simulink model "snap2_f_200msps_64i_4096c_test"  (R2019a)
settings: Solver=VariableStepDiscrete  StartTime=0.0  StopTime=10.0  RelTol=1e-3
libraries: xbsIndex_r4 x8040, casper_library_misc x13, xps_library x6, casper_library_delays x4, casper_library_sources x4, casper_library_reorder x2
(part 1 of 84)
settings Model: ModifiedComment=jackh -- Sun May 10 19:52:36 2020 -- Version 1.426  Creator=mdexter  LastModifiedBy=jackh
settings Model: ModifiedHistory=|
  | jackh -- Sun May 10 19:52:36 2020 -- Version 1.426
  | 
  | jackh -- Sun May 10 19:42:43 2020 -- Version 1.425
  | 
  | make dest udp port dynamically choosable per-packet
  | 
  | jackh -- Sun May 10 17:04:12 2020 -- Version 1.424
  | 
  | make version 0.1
  | 
  | jackh -- Sun May 10 17:03:03 2020 -- Version 1.423
  | 
  | Reorder pols in chan_reorder block so that pol indexing
  | is pol[n] = nth byte of packet
  | 
  | jackh -- Sun May 10 16:52:32 2020 -- Version 1.422
  | 
  | jackh -- Sun May 10 16:08:00 2020 -- Version 1.421
  | 
  | jackh -- Fri May 08 15:06:38 2020 -- Version 1.420
  | 
  | jackh -- Thu May 07 11:32:09 2020 -- Version 1.419
  | 
  | jackh -- Thu May 07 11:18:16 2020 -- Version 1.418
  | 
  | Remove PFB
  | 
  | jackh -- Tue May 05 14:16:03 2020 -- Version 1.417
  | 
  | Make version 0
  | 
  | jackh -- Tue May 05 14:15:21 2020 -- Version 1.416
  | 
  | replace ADC with zeros
  | 
  | jackh -- Tue May 05 14:14:14 2020 -- Version 1.415
  | 
  | Make test design, which is clocked from sys clock and has no ADC
  | 
  | jackh -- Tue May 05 13:29:10 2020 -- Version 1.414
  | 
  | jackh -- Fri May 01 15:26:24 2020 -- Version 1.413
  | 
  | Use sys_clk for testing
  | 
  | jackh -- Fri May 01 15:14:39 2020 -- Version 1.412
  | 
  | Rename 1Gbe core so it is alphabetically first
  | 
  | jackh -- Fri May 01 15:11:49 2020 -- Version 1.411
  | 
  | jackh -- Fri May 01 11:15:12 2020 -- Version 1.410
  | 
  | Change 40gbe core enable so that software enable state can only change immediately after an EOF
  | 
  | jackh -- Fri Apr 24 17:52:32 2020 -- Version 1.409
  | 
  | jackh -- Fri Apr 24 17:51:51 2020 -- Version 1.408
  | 
  | jackh -- Fri Apr 24 17:50:48 2020 -- Version 1.407
  | 
  | jackh -- Fri Apr 24 17:48:49 2020 -- Version 1.406
  | 
  | make packetizer simpler
  | 
  | jackh -- Fri Apr 24 16:17:31 2020 -- Version 1.405
  | 
  | ass max_delay register to delay core
  | 
  | jackh -- Fri Apr 24 16:14:09 2020 -- Version 1.404
  | 
  | jackh -- Fri Apr 24 16:12:03 2020 -- Version 1.403
  | 
  | update eq_tvg to single bram
  | 
  | jackh -- Fri Apr 24 16:08:40 2020 -- Version 1.402
  | 
  | jackh -- Thu Apr 09 09:24:59 2020 -- Version 1.401
  | 
  | make delays 8k long
  | 
  | jackh -- Mon Mar 30 21:41:54 2020 -- Version 1.400
  | 
  | add 1gbe core
  | 
  | jackh -- Sat Mar 14 14:05:43 2020 -- Version 1.399
  | 
  | jackh -- Wed Feb 19 18:48:51 2020 -- Version 1.398
  | 
  | jackh -- Wed Feb 19 18:31:56 2020 -- Version 1.397
  | 
  | jackh -- Wed Feb 19 18:25:06 2020 -- Version 1.396
  | 
  | jackh -- Wed Feb 19 17:10:23 2020 -- Version 1.395
  | 
  | add back in reorders in pfb (having fixed mlib_devel)
  | 
  | jackh -- Tue Feb 18 17:39:49 2020 -- Version 1.394
  | 
  | 10 bitify
  | 
  | jackh -- Tue Feb 18 17:31:23 2020 -- Version 1.393
  | 
  | update_casper_blocks
  | 
  | jackh -- Fri Jan 24 08:04:16 2020 -- Version 1.392
  | replace ADC with sw regs to try and compile for SNAP2
  | 
  | jackh -- Wed Jan 08 08:41:40 2020 -- Version 1.391
  | 
  | 
  | jackh -- Wed Jan 08 08:26:20 2020 -- Version 1.390
  | 
  | 
  | jackh -- Wed Jan 08 08:24:50 2020 -- Version 1.389
  | 
  | 
  | jackh -- Wed Jan 08 08:23:40 2020 -- Version 1.388
  | 
  | 
  | jackh -- Wed Jan 08 08:22:29 2020 -- Version 1.387
  | update platform to SNAP2
  | 
  | jackh -- Wed Jan 08 08:21:36 2020 -- Version 1.386
  | 
  | 
  | jackh -- Wed Jan 08 08:21:09 2020 -- Version 1.385
  | Update internal cross-corr block
  | 
  | jackh -- Wed Jan 08 07:50:59 2020 -- Version 1.384
  | 
  | 
  | jackh -- Wed Jan 08 07:48:46 2020 -- Version 1.383
  | 
  | 
  | jackh -- Wed Jan 08 07:45:47 2020 -- Version 1.382
  | 
  | 
  | jackh -- Wed Jan 08 07:44:03 2020 -- Version 1.381
  | 
  | 
  | jackh -- Wed Jan 08 07:41:17 2020 -- Version 1.380
  | 
  | 
  | jackh -- Wed Jan 08 07:35:58 2020 -- Version 1.379
  | 
  | 
  | jackh -- Wed Jan 08 07:33:51 2020 -- Version 1.378
  | 
  | 
  | jackh -- Wed Jan 08 07:29:30 2020 -- Version 1.377
  | 
  | 
  | jackh -- Wed Jan 08 07:24:27 2020 -- Version 1.376
  | 1st pass fuilly updated to LWA spec
  | 
  | jackh -- Tue Jan 07 10:50:49 2020 -- Version 1.375
  | 
  | 
  | jackh -- Tue Jan 07 10:38:05 2020 -- Version 1.374
  | EQ tvg & FFT updated for 64 inputs
  | 
  | jackh -- Tue Jan 07 10:18:18 2020 -- Version 1.373
  | 
  | 
  | jackh -- Tue Jan 07 10:12:36 2020 -- Version 1.372
  | update FFT
  | 
  | jackh -- Tue Jan 07 09:22:52 2020 -- Version 1.371
  | update FFT core (currently only doing 1/4 of the necessary work)
  | 
  | jackh -- Tue Jan 07 07:40:39 2020 -- Version 1.370
  | Make 64-input. Only corrected up to FFT inputs
  | 
  | jackh -- Tue Jan 07 06:33:25 2020 -- Version 1.369
  | Save a version for LWA expansion project.
  | 
  | jackh -- Sun Oct 27 09:17:26 2019 -- Version 1.368
  | compiled
  | 
  | jackh -- Sun Oct 27 07:24:12 2019 -- Version 1.367
  | remove registering of reorder outputs
  | 
  | jackh -- Sun Oct 27 07:22:37 2019 -- Version 1.366
  | change input snapshot to snap only one of 3 inputs
  | 
  | jackh -- Sun Oct 27 03:59:18 2019 -- Version 1.365
  | remove some superfluous registers to improve timing.
  | Reduce snapshot in input block from 1k samples to 512
  | 
  | jackh -- Sun Oct 27 01:46:50 2019 -- Version 1.364
  | Fix FFT shift bitwidth bug
  | 
  | FFT core was expecting a 16-bit shift, but only a 12bit value was sliced from the control register
  | 
  | jackh -- Fri Aug 30 09:22:01 2019 -- Version 1.363
  | compiled
  | 
  | jackh -- Thu Aug 29 17:13:27 2019 -- Version 1.362
  | change delay shift reg to 3 bit addr
  | 
  | jackh -- Thu Aug 29 11:33:13 2019 -- Version 1.361
  | corr fixes
  | 
  | jackh -- Thu Aug 29 11:09:21 2019 -- Version 1.360
  | latency fix in eqtvg
  | 
  | jackh -- Thu Aug 29 10:02:04 2019 -- Version 1.359
  | compiled
  | 
  | jackh -- Wed Aug 28 15:31:00 2019 -- Version 1.358
  | bump to version 1.3
  | 
  | jackh -- Wed Aug 28 15:26:18 2019 -- Version 1.357
  | change quantization to saturate.
  | Change coefficients to 16_5 (was 16_6)
  | 
  | jackh -- Wed Aug 28 14:17:28 2019 -- Version 1.356
  | remove debugging snapshots hidden in corr vaccs
  | 
  | jackh -- Fri Aug 23 15:01:55 2019 -- Version 1.355
  | compiled
  | 
  | jackh -- Fri Aug 23 10:43:05 2019 -- Version 1.354
  | add snapshot in input block
  | 
  | jackh -- Thu Aug 22 17:13:50 2019 -- Version 1.353
  | fix to eqtvg ram depths
  | 
  | jackh -- Thu Aug 22 15:23:14 2019 -- Version 1.352
  | bump version to 1.2
  | 
  | jackh -- Thu Aug 22 15:22:39 2019 -- Version 1.351
  | Force pairs of pols to have same random number generator to save resources
  | 
  | jackh -- Thu Aug 22 15:19:21 2019 -- Version 1.350
  | rotator channel index counter fixes
  | 
  | eq tvg split bram into 3 (so we can have 6 channels, not 8)
  | 
  | jackh -- Thu Aug 22 12:01:44 2019 -- Version 1.349
  | 
  | 
  | jackh -- Thu Aug 22 12:01:21 2019 -- Version 1.348
  | Changes to rotator precision
  | 
  | jackh -- Tue Aug 20 19:46:09 2019 -- Version 1.347
  | compiled
  | 
  | jackh -- Tue Aug 20 16:55:38 2019 -- Version 1.346
  | increase minimum walsh period to 2**18 fpga clocks (was 2**13)
  | 
  | jackh -- Tue Aug 20 16:40:34 2019 -- Version 1.345
  | 
  | 
  | jackh -- Tue Aug 20 16:15:18 2019 -- Version 1.344
  | bump version to 1.1
  | 
  | jackh -- Tue Aug 20 16:14:49 2019 -- Version 1.343
  | add global enables to phase switch mod/demod to make software easier
  | 
  | jackh -- Mon Aug 19 17:54:23 2019 -- Version 1.342
  | compiled
  | 
  | jackh -- Thu Aug 01 11:53:22 2019 -- Version 1.341
  | make programmable sync delay tolerate delay=0
  | 
  | jackh -- Wed Jul 31 13:49:54 2019 -- Version 1.340
  | comment out corr->rms
  | 
  | jackh -- Mon Jul 29 17:05:34 2019 -- Version 1.339
  | delete corr rms block (not currently enough ram)
  | 
  | jackh -- Mon Jul 29 17:03:29 2019 -- Version 1.338
  | Add version block
  | 
  | jackh -- Mon Jul 29 16:58:22 2019 -- Version 1.337
  | make sync in have a programmable delay
  | Solves 2 problems:
  | 
  | 1) Can start integrations at arbitrary times (good for LST alignment)
  | 2) Can start a 16 second integration chunk on an arbitrary time boundary (needed to avoid the downstream correlator having 16 second start / stop granularity)
  | 
  | jackh -- Mon Jul 29 16:50:03 2019 -- Version 1.336
  | update phasor to 24-bits
  | 
  | jackh -- Sat May 11 17:48:41 2019 -- Version 1.335
  | 
  | 
  | jackh -- Sat May 11 17:46:07 2019 -- Version 1.334
  | 
  | 
  | jackh -- Sat May 11 17:45:44 2019 -- Version 1.333
  | 
  | 
  | jackh -- Sat May 11 17:40:04 2019 -- Version 1.332
  | 
  | 
  | jackh -- Sat May 11 17:36:59 2019 -- Version 1.331
  | add vacc for autocorrs @ 16 bit resolution
  | 
  | deepthi -- Sun Oct 28 15:16:19 2018 -- Version 1.330
  | 
  | 
  | deepthi -- Sat Oct 27 18:45:54 2018 -- Version 1.329
  | 
  | packetizer: Added an 'and' block that holds new_packet signal in high until the first sync.
  | 
  | deepthi -- Sat Oct 27 17:33:32 2018 -- Version 1.328
  | 
  | 1. Change edge_detect location in sync block
  | 
  | deepthi -- Sat Oct 20 22:13:43 2018 -- Version 1.327
  | 
  | 1. Add edge detect to software reg and gpio input in sync block.
  | 
  | 2. Add new corr block with max hold functionality.
  | 
  | jackh -- Tue Oct 09 20:34:13 2018 -- Version 1.326
  | recompile with pmbus_alert register
  | 
  | jackh -- Thu Jul 12 10:55:28 2018 -- Version 1.325
  | 
  | 
  | jackh -- Wed Jul 11 17:20:51 2018 -- Version 1.324
  | syntax
  | 
  | jackh -- Wed Jul 11 17:16:24 2018 -- Version 1.323
  | increase resolution of phase rotator bram.
  | 
  | jackh -- Wed Jul 11 17:10:41 2018 -- Version 1.322
  | 
  | 
  | jackh -- Tue Jul 10 16:08:30 2018 -- Version 1.321
  | scramble rotator channel multiplers to match PFB output order (hopefully)
  | 
  | jackh -- Tue Jul 10 15:51:56 2018 -- Version 1.320
  | 
  | 
  | jackh -- Tue Jul 10 13:37:24 2018 -- Version 1.319
  | fix off-by-one in slicing of mcnt counter, which was having the effect of duplicating mcnts in headers
  | 
  | jackh -- Sat Jul 07 14:17:05 2018 -- Version 1.318
  | compiled
  | 
  | jackh -- Fri Jul 06 10:33:47 2018 -- Version 1.317
  | fix bitbashing to rotator phase addresses
  | 
  | jackh -- Fri Jul 06 10:17:15 2018 -- Version 1.316
  | Add mux to enable / disable rotator
  | 
  | jackh -- Thu Jul 05 17:21:10 2018 -- Version 1.315
  | make some delays behavioural
  | 
  | jackh -- Thu Jul 05 14:48:28 2018 -- Version 1.314
  | 
  | 
  | jackh -- Thu Jul 05 14:46:13 2018 -- Version 1.313
  | 
  | 
  | jackh -- Thu Jul 05 14:43:36 2018 -- Version 1.312
  | 
  | 
  | jackh -- Thu Jul 05 14:40:00 2018 -- Version 1.311
  | 
  | 
  | jackh -- Thu Jul 05 14:36:19 2018 -- Version 1.310
  | 
  | 
  | jackh -- Thu Jul 05 14:26:16 2018 -- Version 1.309
  | integrate rotator into pipeline
  | 
  | jackh -- Thu Jul 05 14:20:20 2018 -- Version 1.308
  | 
  | create phase-rotation block
  | 
  | deepthi -- Thu Jun 07 09:24:03 2018 -- Version 1.307
  | 
  | Replaced the corr block.
  | 
  | deepthi -- Wed Jun 06 12:07:26 2018 -- Version 1.306
  | 
  | 
  | deepthi -- Tue Jun 05 17:46:17 2018 -- Version 1.305
  | 
  | Replaced the corr block with the tested version
  | 
  | deepthi -- Sat May 12 19:11:02 2018 -- Version 1.304
  | 
  | Changed time counter to increment between even/odd banks
  | 
  | deepthi -- Sat May 12 19:06:34 2018 -- Version 1.303
  | 
  | changed timing of eof, valid, data and headers
  | 
  | deepthi -- Mon May 07 23:03:07 2018 -- Version 1.302
  | 
  | 
  | deepthi -- Mon May 07 00:31:44 2018 -- Version 1.301
  | 
  | 
  | deepthi -- Fri May 04 20:13:43 2018 -- Version 1.300
  | 
  | Reduced width sliced from time_ctr
  | 
  | deepthi -- Fri May 04 19:47:57 2018 -- Version 1.299
  | 
  | Added delay to header and ip signals to account for pulse_ext on valid.
  | 
  | deepthi -- Fri May 04 19:23:23 2018 -- Version 1.298
  | 
  | 
  | deepthi -- Thu May 03 16:58:39 2018 -- Version 1.297
  | 
  | 1. Added delays to eof and dest_ip  to account for pulse_ext in valid.
  | 
  | 2. Changed eth_sw expected packet length to include header.
  | 
  | jackh -- Tue May 01 20:38:09 2018 -- Version 1.296
  | compiled
  | 
  | jackh -- Tue May 01 17:49:38 2018 -- Version 1.295
  | Fix to packetizer valid generation, to take into account the 3 (one per antenna) blocks of valid data in each stream of 512 channels
  | 
  | jackh -- Tue May 01 16:49:02 2018 -- Version 1.294
  | make channel selection bram 32-bits wide.
  | 
  | Remove GPU-packing mux / swreg
  | 
  | jackh -- Tue May 01 14:24:16 2018 -- Version 1.293
  | 
  | 
  | jackh -- Tue May 01 14:20:01 2018 -- Version 1.292
  | update chan reorderer
  | 
  | jackh -- Tue May 01 11:43:41 2018 -- Version 1.291
  | compiled
  | 
  | jackh -- Tue May 01 09:44:03 2018 -- Version 1.290
  | 
  | 
  | jackh -- Tue May 01 09:43:34 2018 -- Version 1.289
  | use bram for eq fft descramble map
  | 
  | jackh -- Tue May 01 09:40:26 2018 -- Version 1.288
  | change architecture of corr block -- now stores desired antennas in bram, rather than using a delay tree
  | 
  | jackh -- Mon Apr 30 20:21:35 2018 -- Version 1.287
  | 
  | 
  | jackh -- Mon Apr 30 20:18:20 2018 -- Version 1.286
  | 
  | 
  | jackh -- Mon Apr 30 20:15:51 2018 -- Version 1.285
  | compensate for FFT scrambling in EQ block. Descramble FFT post-requantization in this block
  | 
  | jackh -- Mon Apr 30 19:27:42 2018 -- Version 1.284
  | plausibility pass on corr block
  | 
  | jackh -- Mon Apr 30 12:16:47 2018 -- Version 1.283
  | 
  | 
  | jackh -- Mon Apr 30 12:14:25 2018 -- Version 1.282
  | store chan_reorder reorder map in bram
  | 
  | jackh -- Mon Apr 30 12:05:02 2018 -- Version 1.281
  | remove per-antenna histograms -- now get one histogram with multiplexed input
  | 
  | jackh -- Sun Apr 29 15:50:16 2018 -- Version 1.280
  | 
  | 
  | jackh -- Sun Apr 29 15:37:38 2018 -- Version 1.279
  | 
  | 
  | jackh -- Sun Apr 29 15:27:38 2018 -- Version 1.278
  | First pass packetizer. Regenerate pfb with parameter for serial block inputs
  | 
  | jackh -- Sat Mar 03 12:52:57 2018 -- Version 1.277
  | 
  | 
  | jackh -- Sun Feb 25 12:27:48 2018 -- Version 1.276
  | add pre-pfb reorder
  | 
  | jackh -- Sat Feb 24 13:39:06 2018 -- Version 1.275
  | 
  | jackh -- Sat Feb 24 13:38:40 2018 -- Version 1.274
  | update pfb to 16 inputs
  | 
  | jackh -- Fri Feb 23 18:44:26 2018 -- Version 1.273
  | 
  | 
  | jackh -- Fri Feb 23 18:38:20 2018 -- Version 1.272
  | 
  | 
  | jackh -- Fri Feb 23 17:01:30 2018 -- Version 1.271
  | make fft 8 parallel input
  | 
  | jackh -- Sat Feb 10 13:53:12 2018 -- Version 1.270
  | 
  | 
  | jackh -- Sat Feb 10 13:50:10 2018 -- Version 1.269
  | 
  | 
  | jackh -- Sat Feb 10 13:48:56 2018 -- Version 1.268
  | remove fft preshift
  | 
  | jackh -- Sat Feb 10 13:47:39 2018 -- Version 1.267
  | 
  | 
  | jackh -- Sat Feb 10 13:44:29 2018 -- Version 1.266
  | 
  | 
  | jackh -- Sat Feb 10 13:43:22 2018 -- Version 1.265
  | make delayer dual-pol
  | 
  | jackh -- Sat Feb 10 13:40:59 2018 -- Version 1.264
  | first pass new packet format with no time-based corner turn
  | 
  | jackh -- Fri Feb 09 17:29:05 2018 -- Version 1.263
  | 
  | 
  | jackh -- Fri Feb 09 15:23:03 2018 -- Version 1.262
  | first pass turning everything to 8192 channels
  | 
  | Changed the ants addr to be driven by the same signal that drives chans, ips (used to be driven by ant_tracker).
  | 
  | Removed nants software register that was previously thought to control time stamps (but didn't really)
  | 
  | deepthi -- Wed Jan 31 18:20:45 2018 -- Version 1.261
  | 
  | deepthi -- Mon Jan 29 17:20:36 2018 -- Version 1.260
  | 
  | 
  | deepthi -- Mon Jan 29 17:18:54 2018 -- Version 1.259
  | 
  | 
  | deepthi -- Mon Jan 29 17:18:33 2018 -- Version 1.258
  | 
  | 
  | deepthi -- Mon Jan 29 16:51:19 2018 -- Version 1.257
  | 
  | 
  | deepthi -- Mon Jan 29 16:46:46 2018 -- Version 1.256
  | 
  | 
  | deepthi -- Mon Jan 29 16:37:32 2018 -- Version 1.255
  | 
  | 
  | deepthi -- Mon Jan 29 16:11:03 2018 -- Version 1.254
  | 
  | 
  | deepthi -- Mon Jan 29 15:55:33 2018 -- Version 1.253
  | 
  | 
  | jackh -- Fri Nov 17 19:04:05 2017 -- Version 1.252
  | compiled
  | 
  | jackh -- Wed Nov 15 11:31:03 2017 -- Version 1.251
  | go to 3 corr blocks
  | 
  | jackh -- Tue Nov 14 16:10:40 2017 -- Version 1.250
  | 
  | 
  | jackh -- Tue Nov 14 15:28:37 2017 -- Version 1.249
  | reduce bram use in histogram shared brams
  | 
  | jackh -- Mon Nov 13 18:55:18 2017 -- Version 1.248
  | fix bug in histogram shared bram addr width
  | 
  | jackh -- Fri Nov 10 17:05:56 2017 -- Version 1.247
  | add 4 independent corr subsystems. Add EQ clipping counters
  | 
  | jackh -- Fri Nov 10 14:21:14 2017 -- Version 1.246
  | 
  | 
  | jackh -- Fri Nov 10 14:19:27 2017 -- Version 1.245
  | 
  | 
  | jackh -- Fri Nov 10 11:40:47 2017 -- Version 1.244
  | update to histograms v2
  | 
  | jackh -- Tue Nov 07 22:23:59 2017 -- Version 1.243
  | compiled -- passes eqtvg
  | 
  | jackh -- Tue Nov 07 20:41:00 2017 -- Version 1.242
  | 
  | 
  | jackh -- Tue Nov 07 20:39:30 2017 -- Version 1.241
  | packet header generation fixes
  | 
  | jackh -- Tue Nov 07 17:19:53 2017 -- Version 1.240
  | 
  | 
  | jackh -- Tue Nov 07 17:14:47 2017 -- Version 1.239
  | 
  | 
  | jackh -- Tue Nov 07 17:08:29 2017 -- Version 1.238
  | remove some chan_reorder debug snapshots
  | 
  | jackh -- Tue Nov 07 17:06:39 2017 -- Version 1.237
  | update ps GPIO pins
  | 
  | **** Change packetizer header blocks to can have a separate antenna / ip / chan for each packet. This is for the nants > 3 simulation modes. This will break previous versions of software *****
  | 
  | jackh -- Mon Nov 06 22:06:03 2017 -- Version 1.236
  | add comment to corr_acc_len
  | 
  | Compiled -- passes EQTVG test!
  | 
  | jackh -- Mon Nov 06 15:24:31 2017 -- Version 1.235
  | add OR block in mrst generator so that counter is enabled if/when an arm signal comes
  | 
  | jackh -- Sun Nov 05 21:39:25 2017 -- Version 1.234
  | comment on sync period
  | 
  | jackh -- Sun Nov 05 17:39:01 2017 -- Version 1.233
  | fix bitbasher in 32-spectra corner turn
  | 
  | jackh -- Sun Nov 05 17:05:17 2017 -- Version 1.232
  | aesthetic
  | 
  | jackh -- Sun Nov 05 17:02:53 2017 -- Version 1.231
  | changes to comments
  | 
  | jackh -- Sun Nov 05 17:01:27 2017 -- Version 1.230
  | make acc_len it's own register so we can acc to 2**32
  | 
  | jackh -- Sun Nov 05 16:58:57 2017 -- Version 1.229
  | 
  | 
  | jackh -- Sun Nov 05 16:56:52 2017 -- Version 1.228
  | add internal correlator
  | 
  | jackh -- Sun Nov 05 16:24:21 2017 -- Version 1.227
  | compiled.
  | 
  | jackh -- Sun Nov 05 15:19:13 2017 -- Version 1.226
  | latency tweak to data line in packetizer
  | 
  | jackh -- Sat Nov 04 20:21:54 2017 -- Version 1.225
  | change ethernet debug counters to 32 bits
  | 
  | jackh -- Sat Nov 04 20:05:10 2017 -- Version 1.224
  | make chan reorder map bram 32 bits to aid with software
  | 
  | jackh -- Sat Nov 04 19:51:25 2017 -- Version 1.223
  | change header brams to be 32-bit wide for all values.
  | This makes it easier to deal with the software, which can only write 32-bit bounded words.
  | 
  | jackh -- Sat Nov 04 14:23:39 2017 -- Version 1.222
  | replace big distributed ram in 16-spectra corner turn
  | with simple bit basher manipulation. The distributed ram tool a ridiculous amount of time to synthesize. Hopefully this will be faster.
  | 
  | jackh -- Fri Nov 03 16:25:40 2017 -- Version 1.221
  | 
  | 
  | jackh -- Fri Nov 03 16:17:13 2017 -- Version 1.220
  | update casper blocks on phase switch subsys
  | 
  | jackh -- Fri Nov 03 16:14:34 2017 -- Version 1.219
  | 
  | 
  | jackh -- Fri Nov 03 13:09:23 2017 -- Version 1.218
  | add phase switching and i2c control
  | 
  | jackh -- Fri Nov 03 12:43:29 2017 -- Version 1.217
  | 
  | add i2C controllers
  | 
  | jackh -- Mon Oct 23 16:15:14 2017 -- Version 1.216
  | Add back in Deepthi's fix from f3b63dae07d62
  | 
  | jackh -- Mon Oct 23 16:04:59 2017 -- Version 1.215
  | 
  | 
  | jackh -- Mon Oct 23 14:44:02 2017 -- Version 1.214
  | compiled. Still minor timing errors in the histograms
  | 
  | jackh -- Mon Oct 23 10:40:37 2017 -- Version 1.213
  | change EQ coeffs to one-per channel. Make format 16_6 (was 18_7)
  | 
  | jackh -- Mon Oct 09 15:00:17 2017 -- Version 1.212
  | 
  | halve number of brams in histogram readout
  | 
  | jackh -- Wed Sep 13 11:46:17 2017 -- Version 1.211
  | use built-in tge status regs
  | 
  | jackh -- Tue Sep 12 21:14:25 2017 -- Version 1.210
  | 
  | 
  | jackh -- Tue Sep 12 21:10:57 2017 -- Version 1.209
  | update_casper_blocks(bdroot)
  | 
  | jackh -- Tue Sep 12 21:02:11 2017 -- Version 1.208
  | add histogram to adc stats
  | 
  | jackh -- Fri Jul 14 11:30:38 2017 -- Version 1.207
  | set map = reord_map in chan_reorder blocks which use matlab scripts to generate their reorders.
  | 
  | jackh -- Thu Jul 13 17:48:05 2017 -- Version 1.206
  | change sync period to a 32-bit sw reg (was hardcoded 9! * 1024)
  | 
  | deepthi -- Thu Jul 13 13:07:36 2017 -- Version 1.205
  | 
  | 
  | deepthi -- Thu Jul 13 12:10:35 2017 -- Version 1.204
  | 
  | 
  | deepthi -- Wed Jul 12 16:52:46 2017 -- Version 1.203
  | 
  | 
  | deepthi -- Wed Jul 12 15:57:48 2017 -- Version 1.202
  | 
  | 
  | deepthi -- Tue Jul 11 19:00:41 2017 -- Version 1.201
  | 
  | 
  | deepthi -- Tue Jul 11 18:54:05 2017 -- Version 1.200
  | 
  | 
  | deepthi -- Tue Jul 11 18:52:32 2017 -- Version 1.199
  | 
  | 
  | deepthi -- Mon Jul 10 16:18:51 2017 -- Version 1.198
  | 
  | 
  | deepthi -- Sun Jul 09 18:15:02 2017 -- Version 1.197
  | 
  | 
  | deepthi -- Thu Jul 06 13:54:16 2017 -- Version 1.196
  | 
  | 
  | jackh -- Mon Jul 03 11:01:40 2017 -- Version 1.195
  | 
  | 
  | jackh -- Fri Jun 30 13:59:17 2017 -- Version 1.194
  | enable CPU tx/rx buffer on tge core. Needed for microblaze.
  | 
  | jackh -- Mon Jun 26 11:33:24 2017 -- Version 1.193
  | 
  | 
  | jackh -- Thu Jun 22 14:37:16 2017 -- Version 1.192
  | add history prompting
settings DataIOCC: LimitDataPoints=on  SaveFormat=Array  SignalLoggingSaveFormat=ModelDataLogs  ReturnWorkspaceOutputs=off
settings OptimizationCC: DefaultParameterBehavior=Inlined  ExpressionDepthLimit=2147483647  LifeSpan=inf
settings DebuggingCC: UnderspecifiedInitializationDetection=Classic  MergeDetectMultiDrivingBlocksExec=none  SolverPrmCheckMsg=warning  FcnCallInpInsideContextMsg=warning  AllowSymbolicDim=off  StateNameClashWarn=warning  SFUnexpectedBacktrackingDiag=warning  SFNoUnconditionalDefaultTransitionDiag=warning  SFExecutionAtInitializationDiag=none  ArithmeticOperatorsInVariantConditions=warning
settings HardwareCC: ProdBitPerPointer=32  ProdBitPerSizeT=32  ProdBitPerPtrDiffT=32  ProdLargestAtomicFloat=None  ProdIntDivRoundTo=Undefined  ProdEndianess=Unspecified  ProdWordSize=32  ProdHWDeviceType=32-bit Generic
settings ModelReferenceCC: PropagateSignalLabelsOutOfModel=off
settings SFSimCC: SimUseLocalCustomCode=off
settings RTWCC: RTWUseLocalCustomCode=off
settings CodeAppCC: StateflowObjectComments=on
settings GRTTargetCC: TargetLangStandard=C89/C90 (ANSI)  GeneratePreprocessorConditionals=Disable all  CombineOutputUpdateFcns=off  GRTInterface=on
settings ConfigComp: CovMetricSettings=dw  CovHtmlReporting=on  CovSaveCumulativeToWorkspaceVar=on  CovSaveSingleToWorkspaceVar=on  CovExternalEMLEnable=off

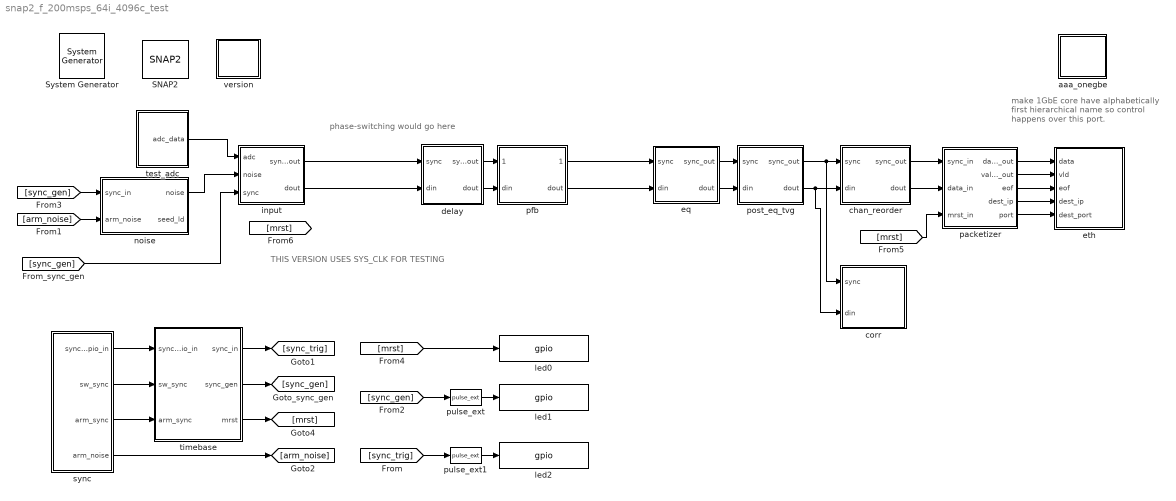
== system snap2_f_200msps_64i_4096c_test ==
  note: THIS VERSION USES SYS_CLK FOR TESTING
  note: make 1GbE core have alphabetically
      | first hierarchical name so control
      | happens over this port.
  note: phase-switching
      | would go here
  " System Generator" : xbsIndex_r4/ System Generator  Tag=genX  xilinxfamily=kintexu  part=xcku115  speed=-2-e  package=flvf1924  synthesis_tool=XST  clock_wrapper=Clock Enables  directory=/home/jackh/src/caltech-lwa/snap2_f_200msps_64i_4096c_test/sysgen  proj_type=Vivado  Synth_file=Vivado Synthesis Defaults  Impl_file=Vivado Implementation Defaults  testbench=off  simulink_period=1  sysclk_period=10  dcm_input_clock_period=10  incr_netlist=off  trim_vbits=Everywhere in SubSystem  dbl_ovrd=According to Block Masks  core_generation=According to Block Masks  run_coregen=off  deprecated_control=off  eval_field=0  block_type=sysgen
  SNAP2 : xps_library/Platforms/SNAP2  Tag=xps:xsg  hw_sys=SNAP2:xcku115  clk_src=sys_clk  clk_rate=100  use_microblaze=on  sample_period=1  synthesis_tool=XST
      settings: SourceProductName=CASPER XPS Blockset
  aaa_onegbe : Subsystem
  chan_reorder : Subsystem
  corr : Subsystem
  delay : Subsystem
  eq : Subsystem
  eth : Subsystem
  input : Subsystem
  led0 : xps_library/IO/gpio  Tag=xps:gpio  io_group_params_forwarded=on  io_group=ROACH2:led  io_group_real=led  io_group_custom=0  io_dir=out  arith_type=Boolean  bitwidth=1  bin_pt=0  bit_index=0  sample_period=1  use_single_ended=off  use_ddr=off  reg_iob=on  reg_clk_phase=0  termination=None
      settings: SourceProductName=CASPER XPS Blockset
  led1 : xps_library/IO/gpio  Tag=xps:gpio  io_group_params_forwarded=on  io_group=ROACH2:led  io_group_real=led  io_group_custom=0  io_dir=out  arith_type=Boolean  bitwidth=1  bin_pt=0  bit_index=1  sample_period=1  use_single_ended=off  use_ddr=off  reg_iob=on  reg_clk_phase=0  termination=None
      settings: SourceProductName=CASPER XPS Blockset
  led2 : xps_library/IO/gpio  Tag=xps:gpio  io_group_params_forwarded=on  io_group=ROACH2:led  io_group_real=led  io_group_custom=0  io_dir=out  arith_type=Boolean  bitwidth=1  bin_pt=0  bit_index=2  sample_period=1  use_single_ended=off  use_ddr=off  reg_iob=on  reg_clk_phase=0  termination=None
      settings: SourceProductName=CASPER XPS Blockset
  noise : Subsystem
  packetizer : Subsystem  mask{nchan_bits=12, npol_bits=6, nparallel_bits=5}
      mask prompts: nchan_bits "Number of channels (including unsent) (2^?)"; npol_bits "Number of pols (2^?)"; nparallel_bits "Parallel samples (2^?)"
  pfb : Subsystem
  post_eq_tvg : Subsystem
  pulse_ext : casper_library_misc/pulse_ext  pulse_len=2^26
      settings: SourceProductName=CASPER DSP Blockset
  pulse_ext1 : casper_library_misc/pulse_ext  pulse_len=2^26
      settings: SourceProductName=CASPER DSP Blockset
  sync : Subsystem
  test_adc : Subsystem
  timebase : Subsystem
  version : Subsystem  mask{ver_maj=0, ver_min=1}
      mask prompts: ver_maj "Major version"; ver_min "Minor version"
  wires:
  test_adc/1(adc_data) -> input/1(adc)
  noise/1(noise) -> input/2(noise)
  sync/1(sync_gpio_in) -> timebase/1(sync_gpio_in)
  sync/2(sw_sync) -> timebase/2(sw_sync)
  sync/3(arm_sync) -> timebase/3(arm_sync)
  [arm_noise] -> noise/2(arm_noise)
  [sync_gen] -> noise/1(sync_in)
  timebase/2(sync_gen) -> [sync_gen]
  timebase/1(sync_in) -> [sync_trig]
  sync/4(arm_noise) -> [arm_noise]
  [sync_gen] -> input/3(sync)
  post_eq_tvg/1(sync_out) -> corr/1(sync), chan_reorder/1(sync)
  post_eq_tvg/2(dout) -> corr/2(din), chan_reorder/2(din)
  timebase/3(mrst) -> [mrst]
  [sync_gen] -> pulse_ext/1
  [mrst] -> led0/1
  pulse_ext/1 -> led1/1
  delay/1(sync_out) -> pfb/1(sync_in)
  delay/2(dout) -> pfb/2(din)
  [sync_trig] -> pulse_ext1/1
  pulse_ext1/1 -> led2/1
  input/2(dout) -> delay/2(din)
  input/1(sync_out) -> delay/1(sync)
  chan_reorder/1(sync_out) -> packetizer/1(sync_in)
  chan_reorder/2(dout) -> packetizer/2(data_in)
  [mrst] -> packetizer/3(mrst_in)
  pfb/1(sync_out) -> eq/1(sync)
  pfb/2(dout) -> eq/2(din)
  eq/1(sync_out) -> post_eq_tvg/1(sync)
  eq/2(dout) -> post_eq_tvg/2(din)
  packetizer/4(dest_ip) -> eth/4(dest_ip)
  packetizer/3(eof) -> eth/3(eof)
  packetizer/1(data_out) -> eth/1(data)
  packetizer/5(port) -> eth/5(dest_port)
  packetizer/2(valid_out) -> eth/2(vld)

== system snap2_f_200msps_64i_4096c_test/aaa_onegbe ==
  Constant : xbsIndex_r4/Constant  const=0  gui_display_data_type=Boolean  arith_type=Boolean  n_bits=16  bin_pt=14  preci_type=Single  exp_width=8  frac_width=24  explicit_period=on  period=1  equ=P=C  opselect=C  inp2=PCIN>>17  opr=+  inp1=P  carry=CIN  dbl_ovrd=off  block_type=constant
  Constant1 : xbsIndex_r4/Constant  const=0  gui_display_data_type=Fixed-point  arith_type=Unsigned  n_bits=8  bin_pt=0  preci_type=Single  exp_width=8  frac_width=24  explicit_period=on  period=1  equ=P=C  opselect=C  inp2=PCIN>>17  opr=+  inp1=P  carry=CIN  dbl_ovrd=off  block_type=constant
  Constant2 : xbsIndex_r4/Constant  const=1  gui_display_data_type=Boolean  arith_type=Boolean  n_bits=16  bin_pt=14  preci_type=Single  exp_width=8  frac_width=24  explicit_period=on  period=1  equ=P=C  opselect=C  inp2=PCIN>>17  opr=+  inp1=P  carry=CIN  dbl_ovrd=off  block_type=constant
  Constant3 : xbsIndex_r4/Constant  const=0  gui_display_data_type=Fixed-point  arith_type=Unsigned  n_bits=32  bin_pt=0  preci_type=Single  exp_width=8  frac_width=24  explicit_period=on  period=1  equ=P=C  opselect=C  inp2=PCIN>>17  opr=+  inp1=P  carry=CIN  dbl_ovrd=off  block_type=constant
  Constant4 : xbsIndex_r4/Constant  const=0  gui_display_data_type=Fixed-point  arith_type=Unsigned  n_bits=16  bin_pt=0  preci_type=Single  exp_width=8  frac_width=24  explicit_period=on  period=1  equ=P=C  opselect=C  inp2=PCIN>>17  opr=+  inp1=P  carry=CIN  dbl_ovrd=off  block_type=constant
  one_GbE : xps_library/IO/one_gbe  Tag=xps:onegbe  local_en=on  dis_cpu_rx=off  dis_cpu_tx=off  cpu_promiscuous=off  local_mac=hex2dec('123456789abc')  local_ip=hex2dec('c0a8290a')  local_port=4321  local_gateway=1
      settings: SourceProductName=CASPER XPS Blockset
  wires:
  Constant/1 -> one_GbE/7, one_GbE/4, one_GbE/2, one_GbE/1
  Constant3/1 -> one_GbE/5
  Constant1/1 -> one_GbE/3
  Constant2/1 -> one_GbE/8
  Constant4/1 -> one_GbE/6

== system snap2_f_200msps_64i_4096c_test/chan_reorder ==
  note: block transpose
      | last two words, so pol order is
      | 0, 1, ..., 31 (first word)
      | 32, 33, ..., 63 (second word)
  note: blockwise transpose:
      |
      | output order is now:
      |
      | chans (512) x pols (2) x chans (8) x pols (32)
      |
      | last axis here is pol:
      | n, n+16, n+32, n+48,
      | n+1, n+17, n+32, n+49, ...
      | ...
      | n+7, n+23, n+39, n+55
  note: Reorder each word:
      |
      | order is now:
      |
      | chans (512) x pols (16) x chans (8) x pols (4)
      |
      | Last index here is pol: n, n+16, n+32, n+48
  note: Input order is:
      |
      | pols (16) x chans (512) x pols (4) x chans (8)
      |
      | Transpose first two axes. Output order is:
      | chans (512) x pols (16) x pols (4) x chans (8)
  note: Use this programmable
      | map to mess with the channel
      | ordering.
      |
      | Out of every block of 128 channels,
      | only the first 80 will be sent.
      | So fold the edges of the band into unwanted slots
      |
      | Input is 8 channels x 4 antennas in parallel.
      | Over 512 clocks we get a full spectrum for these 4 antennas.
      | Over the next 16x512 clocks we get spectra for 64 antennas total
  note: Serial transpose along fastest axes
      |
      | output order is now:
      |
      | chans (512) x chans (8) x pols (2) x pols (32)
  sync : Inport
  din : Inport  Port=2
  Constant : xbsIndex_r4/Constant  const=1  gui_display_data_type=Boolean  arith_type=Boolean  n_bits=1  bin_pt=0  preci_type=Single  exp_width=8  frac_width=24  explicit_period=on  period=1  equ=P=C  opselect=C  inp2=PCIN>>17  opr=+  inp1=P  carry=CIN  dbl_ovrd=off  block_type=constant
  Constant2 : xbsIndex_r4/Constant  const=1  gui_display_data_type=Boolean  arith_type=Boolean  n_bits=1  bin_pt=0  preci_type=Single  exp_width=8  frac_width=24  explicit_period=on  period=1  equ=P=C  opselect=C  inp2=PCIN>>17  opr=+  inp1=P  carry=CIN  dbl_ovrd=off  block_type=constant
  Constant3 : xbsIndex_r4/Constant  const=1  gui_display_data_type=Boolean  arith_type=Boolean  n_bits=1  bin_pt=0  preci_type=Single  exp_width=8  frac_width=24  explicit_period=on  period=1  equ=P=C  opselect=C  inp2=PCIN>>17  opr=+  inp1=P  carry=CIN  dbl_ovrd=off  block_type=constant
  bus_create : Subsystem  AncestorBlock=casper_library_flow_control/bus_create  mask(bus_create){inputNum=8}
      mask prompts: inputNum "Number of inputs:"
      mask init:
      | bus_create_init(gcb,...
      |     'inputNum', inputNum);
  bus_expand2 : Subsystem  AncestorBlock=casper_library_flow_control/bus_expand  mask(bus_expand){mode=divisions of equal size, outputNum=8, outputWidth=4*8, outputBinaryPt=0, outputArithmeticType=0, show_format=off, outputToWorkspace=off, variablePrefix=out, outputToModelAsWell=on}
      mask prompts: outputNum "Number of outputs:"; outputWidth "Output width:"; outputBinaryPt "Output binary point position:"; outputArithmeticType "Output arithmetic type (ufix=0, fix=1, bool=2):"; show_format "Print format string?"; outputToWorkspace "Output to workspace?"; variablePrefix "Variable name prefix:"; outputToModelAsWell "Output to model as well?"
      mask help:
      | Expands a 'bus' made using a bus_create or Xilinx
      | concat block.
      | The input will be divided into the specified number
      | of outputs with the specified arithmetic types.
      | Divisions are made from most significant bit.
      mask init:
      | bus_expand_init(gcb,...
      |     'mode', mode, ...
      |     'outputNum', outputNum, ...
      |     'outputWidth', outputWidth, ...
      |     'outputBinaryPt', outputBinaryPt, ...
      |     'outputArithmeticType', outputArithmeticType, ...
      |     'show_format', show_format, ...
      |     'outputToWorkspace', outputToWorkspace, ...
      |     'variablePrefix', variablePrefix, ...
      |     'outputToModelAsWell', outputToModelAsWell);
      settings: AttributesFormatString=8 outputs
      mask TypeOptions mode: divisions of equal size | divisions of arbitrary size
      mask Callback mode: bus_expand_callback();
      mask Callback outputWidth: bus_expand_callback();
      mask Callback outputToWorkspace: bus_expand_callback();
  dynamic : Subsystem  AncestorBlock=casper_library_reorder/reorder  mask(reorder){map=[0:512-1], n_bits=8*8*4, n_inputs=1, bram_latency=3, map_latency=3, fanout_latency=2, double_buffer=1, bram_map=on, software_controlled=on}
      mask prompts: map "Output Order:"; n_bits "Data width in"; n_inputs "Number of inputs"; bram_latency "BRAM Latency"; map_latency "Map Latency"; fanout_latency "Fanout latency"; double_buffer "Double Buffer"; bram_map "Use BlockRAM for Map"; software_controlled "Use runtime software control"
      mask init:
      | reorder_init(gcb, ...
      |     'map', map, ...
      |     'n_bits', n_bits, ...
      |     'n_inputs', n_inputs, ...
      |     'bram_latency', bram_latency, ...
      |     'map_latency', map_latency, ...
      |     'fanout_latency', fanout_latency, ...
      |     'double_buffer', double_buffer, ...
      |     'bram_map', bram_map, ...
      |     'software_controlled', software_controlled);
      settings: AttributesFormatString=order=2
      mask Help: eval('xlWeb(''http://casper.berkeley.edu/wiki/Reorder'')')
  parallel_reorder : Subsystem
  pol_reorder : Subsystem
  reorder : Subsystem  AncestorBlock=casper_library_reorder/reorder  mask(reorder){map=reshape(reshape([0:8192 - 1], 512, 16)', 1, 8192), n_bits=8*4*8, n_inputs=1, bram_latency=3, map_latency=1, fanout_latency=0, double_buffer=0, bram_map=on, software_controlled=off}
      mask prompts: map "Output Order:"; n_bits "Data width in"; n_inputs "Number of inputs"; bram_latency "BRAM Latency"; map_latency "Map Latency"; fanout_latency "Fanout latency"; double_buffer "Double Buffer"; bram_map "Use BlockRAM for Map"; software_controlled "Use runtime software control"
      mask init: same as snap2_f_200msps_64i_4096c_test/chan_reorder/dynamic
      settings: AttributesFormatString=order=13
      mask Help: eval('xlWeb(''http://casper.berkeley.edu/wiki/Reorder'')')
  reorder2 : Subsystem  AncestorBlock=casper_library_reorder/reorder  mask(reorder){map=reshape(reshape([0:16 - 1], 8, 2)', 1, 16), n_bits=32*8, n_inputs=1, bram_latency=3, map_latency=1, fanout_latency=0, double_buffer=1, bram_map=on, software_controlled=off}
      mask prompts: map "Output Order:"; n_bits "Data width in"; n_inputs "Number of inputs"; bram_latency "BRAM Latency"; map_latency "Map Latency"; fanout_latency "Fanout latency"; double_buffer "Double Buffer"; bram_map "Use BlockRAM for Map"; software_controlled "Use runtime software control"
      mask init: same as snap2_f_200msps_64i_4096c_test/chan_reorder/dynamic
      settings: AttributesFormatString=order=2
      mask Help: eval('xlWeb(''http://casper.berkeley.edu/wiki/Reorder'')')
  square_transposer : Subsystem  AncestorBlock=casper_library_reorder/square_transposer  mask(square_transposer){n_inputs=3, async=off}
      mask prompts: n_inputs "Number of inputs (2^?):"; async "Aynchronus operation"
      mask init:
      | square_transposer_init(gcb,...
      |     'n_inputs', n_inputs, ...
      |     'async', async);
      settings: AttributesFormatString=n_inputs=3
      mask Help: eval('xlWeb(''http://casper.berkeley.edu/wiki/Square_transposer'')')
  sync_out : Outport
  dout : Outport  Port=2
  wires:
  Constant/1 -> reorder/2(en)
  reorder/3(dout0) -> parallel_reorder/1(din)
  Constant2/1 -> dynamic/2(en)
  sync/1 -> dynamic/1(sync)
  din/1 -> dynamic/3(din0)
  dynamic/2(valid) -> ?
  dynamic/3(dout0) -> reorder/3(din0)
  dynamic/1(sync_out) -> reorder/1(sync)
  parallel_reorder/1(dout) -> bus_expand2/1(bus_in)
  reorder/1(sync_out) -> square_transposer/1(sync)
  bus_expand2/4(out5) -> square_transposer/5(in3)
  bus_expand2/7(out2) -> square_transposer/8(in6)
  bus_expand2/1(msb_out8) -> square_transposer/2(in0)
  bus_expand2/2(out7) -> square_transposer/3(in1)
  bus_expand2/6(out3) -> square_transposer/7(in5)
  bus_expand2/3(out6) -> square_transposer/4(in2)
  bus_expand2/5(out4) -> square_transposer/6(in4)
  bus_expand2/8(lsb_out1) -> square_transposer/9(in7)
  square_transposer/1(sync_out) -> reorder2/1(sync)
  square_transposer/9(out7) -> bus_create/8(in8)
  square_transposer/8(out6) -> bus_create/7(in7)
  square_transposer/6(out4) -> bus_create/5(in5)
  square_transposer/7(out5) -> bus_create/6(in6)
  square_transposer/2(out0) -> bus_create/1(in1)
  square_transposer/3(out1) -> bus_create/2(in2)
  square_transposer/4(out2) -> bus_create/3(in3)
  square_transposer/5(out3) -> bus_create/4(in4)
  Constant3/1 -> reorder2/2(en)
  bus_create/1(bus_out) -> reorder2/3(din0)
  reorder2/1(sync_out) -> pol_reorder/1(sync)
  reorder2/3(dout0) -> pol_reorder/2(din)
  pol_reorder/1(sync_out) -> sync_out/1
  pol_reorder/2(dout) -> dout/1

== system snap2_f_200msps_64i_4096c_test/corr ==
  sync : Inport
  din : Inport  Port=2
  0 : Subsystem  mask{nchan_bits=12, npol_bits=4}
      mask prompts: nchan_bits "Number of channels (2^?)"; npol_bits "Number of pols (2^?)"
  wires:
  sync/1 -> 0/1(sync)
  din/1 -> 0/2(din)

== system snap2_f_200msps_64i_4096c_test/delay ==
  sync : Inport
  din : Inport  Port=2
  0 : Subsystem
  1 : Subsystem
  10 : Subsystem
  11 : Subsystem
  12 : Subsystem
  13 : Subsystem
  14 : Subsystem
  15 : Subsystem
  16 : Subsystem
  17 : Subsystem
  18 : Subsystem
  19 : Subsystem
  2 : Subsystem
  20 : Subsystem
  21 : Subsystem
  22 : Subsystem
  23 : Subsystem
  24 : Subsystem
  25 : Subsystem
  26 : Subsystem
  27 : Subsystem
  28 : Subsystem
  29 : Subsystem
  3 : Subsystem
  30 : Subsystem
  31 : Subsystem
  32 : Subsystem
  33 : Subsystem
  34 : Subsystem
  35 : Subsystem
  36 : Subsystem
  37 : Subsystem
  38 : Subsystem
  39 : Subsystem
  4 : Subsystem
  40 : Subsystem
  41 : Subsystem
  42 : Subsystem
  43 : Subsystem
  44 : Subsystem
  45 : Subsystem
  46 : Subsystem
  47 : Subsystem
  48 : Subsystem
  49 : Subsystem
  5 : Subsystem
  50 : Subsystem
  51 : Subsystem
  52 : Subsystem
  53 : Subsystem
  54 : Subsystem
  55 : Subsystem
  56 : Subsystem
  57 : Subsystem
  58 : Subsystem
  59 : Subsystem
  6 : Subsystem
  60 : Subsystem
  61 : Subsystem
  62 : Subsystem
  63 : Subsystem
  7 : Subsystem
  8 : Subsystem
  9 : Subsystem
  Constant : xbsIndex_r4/Constant  const=2^13  gui_display_data_type=Fixed-point  arith_type=Unsigned  n_bits=32  bin_pt=0  preci_type=Single  exp_width=8  frac_width=24  explicit_period=on  period=1  equ=P=C  opselect=C  inp2=PCIN>>17  opr=+  inp1=P  carry=CIN  dbl_ovrd=off  block_type=constant
  bus_create : Subsystem  AncestorBlock=casper_library_flow_control/bus_create  mask(bus_create){inputNum=64}
      mask prompts: inputNum "Number of inputs:"
      mask init:
      | bus_create_init(gcb,...
      |     'inputNum', inputNum);
  bus_expand : Subsystem  AncestorBlock=casper_library_flow_control/bus_expand  mask(bus_expand){mode=divisions of equal size, outputNum=8*8, outputWidth=10, outputBinaryPt=0, outputArithmeticType=0, show_format=off, outputToWorkspace=off, variablePrefix=out, outputToModelAsWell=on}
      mask prompts: outputNum "Number of outputs:"; outputWidth "Output width:"; outputBinaryPt "Output binary point position:"; outputArithmeticType "Output arithmetic type (ufix=0, fix=1, bool=2):"; show_format "Print format string?"; outputToWorkspace "Output to workspace?"; variablePrefix "Variable name prefix:"; outputToModelAsWell "Output to model as well?"
      mask help:
      | Expands a 'bus' made using a bus_create or Xilinx
      | concat block.
      | The input will be divided into the specified number
      | of outputs with the specified arithmetic types.
      | Divisions are made from most significant bit.
      mask init: same as snap2_f_200msps_64i_4096c_test/chan_reorder/bus_expand2
      settings: AttributesFormatString=64 outputs
      mask TypeOptions mode: divisions of equal size | divisions of arbitrary size
      mask Callback mode: bus_expand_callback();
      mask Callback outputWidth: bus_expand_callback();
      mask Callback outputToWorkspace: bus_expand_callback();
  max_delay : Subsystem  Tag=xps:sw_reg  AncestorBlock=xps_library/Memory/software_register  mask(swreg){io_dir=To Processor, io_delay=0, init_val=0, sample_period=1, names=reg, bitwidths=32, bin_pts=0, arith_types=0, sim_port=on, show_format=off}
      mask prompts: io_dir "I/O direction"; io_delay "I/O delay"; init_val "Initial Value"; sample_period "Sample period"; names "Bitfield names [msb...lsb]"; bitwidths "Bitfield widths"; bin_pts "Bitfield binary pts"; arith_types "Bitfield types, ufix=0, fix=1, bool=2"; sim_port "Provide sim input/output?"; show_format "Print format string?"
      mask help: A 32-bit software-accessible register. Can be divided into bitfields of varying widths and types using the fields in the block mask.
      mask init:
      | swreg_init(gcb)
      settings: AttributesFormatString=1output
      mask TypeOptions io_dir: To Processor | From Processor
      mask Callback io_dir:
      | mask_enables = get_param(gcb, 'MaskEnables');
      | mask_names = get_param(gcb, 'MaskNames');
      | if strcmp(get_param(gcb, 'io_dir'), 'To Processor'),
      |     mask_enables{ismember(mask_names, 'sample_period')} = 'off';
      | else
      |     mask_enables{ismember(mask_names, 'sample_period')} = 'on';
      | end
      | set_param(gcb, 'MaskEnables', mask_enables);
      mask DialogControl ParameterTabVar0 Prompt: Setup
  sync_out : Outport
  dout : Outport  Port=2
  wires:
  sync/1 -> sync_out/1
  din/1 -> bus_expand/1(bus_in)
  bus_expand/1(msb_out64) -> 0/1(din)
  bus_expand/2(out63) -> 1/1(din)
  bus_expand/3(out62) -> 2/1(din)
  bus_expand/4(out61) -> 3/1(din)
  bus_expand/5(out60) -> 4/1(din)
  bus_expand/6(out59) -> 5/1(din)
  bus_expand/7(out58) -> 6/1(din)
  bus_expand/8(out57) -> 7/1(din)
  bus_expand/9(out56) -> 8/1(din)
  bus_expand/10(out55) -> 9/1(din)
  bus_expand/11(out54) -> 10/1(din)
  bus_expand/12(out53) -> 11/1(din)
  bus_expand/13(out52) -> 12/1(din)
  bus_expand/14(out51) -> 13/1(din)
  bus_expand/15(out50) -> 14/1(din)
  bus_expand/16(out49) -> 15/1(din)
  bus_expand/17(out48) -> 16/1(din)
  bus_expand/18(out47) -> 17/1(din)
  bus_expand/19(out46) -> 18/1(din)
  bus_expand/20(out45) -> 19/1(din)
  bus_expand/21(out44) -> 20/1(din)
  bus_expand/22(out43) -> 21/1(din)
  bus_expand/23(out42) -> 22/1(din)
  bus_expand/24(out41) -> 23/1(din)
  bus_expand/25(out40) -> 24/1(din)
  bus_expand/26(out39) -> 25/1(din)
  bus_expand/27(out38) -> 26/1(din)
  bus_expand/28(out37) -> 27/1(din)
  bus_expand/29(out36) -> 28/1(din)
  bus_expand/30(out35) -> 29/1(din)
  bus_expand/31(out34) -> 30/1(din)
  bus_expand/32(out33) -> 31/1(din)
  bus_expand/33(out32) -> 32/1(din)
  bus_expand/34(out31) -> 33/1(din)
  bus_expand/35(out30) -> 34/1(din)
  bus_expand/36(out29) -> 35/1(din)
  bus_expand/37(out28) -> 36/1(din)
  bus_expand/38(out27) -> 37/1(din)
  bus_expand/39(out26) -> 38/1(din)
  bus_expand/40(out25) -> 39/1(din)
  bus_expand/41(out24) -> 40/1(din)
  bus_expand/42(out23) -> 41/1(din)
  bus_expand/43(out22) -> 42/1(din)
  bus_expand/44(out21) -> 43/1(din)
  bus_expand/45(out20) -> 44/1(din)
  bus_expand/46(out19) -> 45/1(din)
  bus_expand/47(out18) -> 46/1(din)
  bus_expand/48(out17) -> 47/1(din)
  bus_expand/49(out16) -> 48/1(din)
  bus_expand/50(out15) -> 49/1(din)
  bus_expand/51(out14) -> 50/1(din)
  bus_expand/52(out13) -> 51/1(din)
  bus_expand/53(out12) -> 52/1(din)
  bus_expand/54(out11) -> 53/1(din)
  bus_expand/55(out10) -> 54/1(din)
  bus_expand/56(out9) -> 55/1(din)
  bus_expand/57(out8) -> 56/1(din)
  bus_expand/58(out7) -> 57/1(din)
  bus_expand/59(out6) -> 58/1(din)
  bus_expand/60(out5) -> 59/1(din)
  bus_expand/61(out4) -> 60/1(din)
  bus_expand/62(out3) -> 61/1(din)
  bus_expand/63(out2) -> 62/1(din)
  bus_expand/64(lsb_out1) -> 63/1(din)
  0/1(dout) -> bus_create/1(in1)
  1/1(dout) -> bus_create/2(in2)
  2/1(dout) -> bus_create/3(in3)
  3/1(dout) -> bus_create/4(in4)
  4/1(dout) -> bus_create/5(in5)
  5/1(dout) -> bus_create/6(in6)
  6/1(dout) -> bus_create/7(in7)
  7/1(dout) -> bus_create/8(in8)
  8/1(dout) -> bus_create/9(in9)
  9/1(dout) -> bus_create/10(in10)
  10/1(dout) -> bus_create/11(in11)
  11/1(dout) -> bus_create/12(in12)
  12/1(dout) -> bus_create/13(in13)
  13/1(dout) -> bus_create/14(in14)
  14/1(dout) -> bus_create/15(in15)
  15/1(dout) -> bus_create/16(in16)
  16/1(dout) -> bus_create/17(in17)
  17/1(dout) -> bus_create/18(in18)
  18/1(dout) -> bus_create/19(in19)
  19/1(dout) -> bus_create/20(in20)
  20/1(dout) -> bus_create/21(in21)
  21/1(dout) -> bus_create/22(in22)
  22/1(dout) -> bus_create/23(in23)
  23/1(dout) -> bus_create/24(in24)
  24/1(dout) -> bus_create/25(in25)
  25/1(dout) -> bus_create/26(in26)
  26/1(dout) -> bus_create/27(in27)
  27/1(dout) -> bus_create/28(in28)
  28/1(dout) -> bus_create/29(in29)
  29/1(dout) -> bus_create/30(in30)
  30/1(dout) -> bus_create/31(in31)
  31/1(dout) -> bus_create/32(in32)
  32/1(dout) -> bus_create/33(in33)
  33/1(dout) -> bus_create/34(in34)
  34/1(dout) -> bus_create/35(in35)
  35/1(dout) -> bus_create/36(in36)
  36/1(dout) -> bus_create/37(in37)
  37/1(dout) -> bus_create/38(in38)
  38/1(dout) -> bus_create/39(in39)
  39/1(dout) -> bus_create/40(in40)
  40/1(dout) -> bus_create/41(in41)
  41/1(dout) -> bus_create/42(in42)
  42/1(dout) -> bus_create/43(in43)
  43/1(dout) -> bus_create/44(in44)
  44/1(dout) -> bus_create/45(in45)
  45/1(dout) -> bus_create/46(in46)
  46/1(dout) -> bus_create/47(in47)
  47/1(dout) -> bus_create/48(in48)
  48/1(dout) -> bus_create/49(in49)
  49/1(dout) -> bus_create/50(in50)
  50/1(dout) -> bus_create/51(in51)
  51/1(dout) -> bus_create/52(in52)
  52/1(dout) -> bus_create/53(in53)
  53/1(dout) -> bus_create/54(in54)
  54/1(dout) -> bus_create/55(in55)
  55/1(dout) -> bus_create/56(in56)
  56/1(dout) -> bus_create/57(in57)
  57/1(dout) -> bus_create/58(in58)
  58/1(dout) -> bus_create/59(in59)
  59/1(dout) -> bus_create/60(in60)
  60/1(dout) -> bus_create/61(in61)
  61/1(dout) -> bus_create/62(in62)
  62/1(dout) -> bus_create/63(in63)
  63/1(dout) -> bus_create/64(in64)
  bus_create/1(bus_out) -> dout/1
  Constant/1 -> max_delay/1(out_reg)
